simulink model "reglareperturbatie"  (R2016a)
settings: Solver=ode4  StartTime=0.0  StopTime=2000  FixedStep=0.01  RelTol=1e-3
undefined symbols (not defined in the file): k, k2, keta
libraries: simulink x1
settings Model: Creator=Danut  LastModifiedBy=Danut

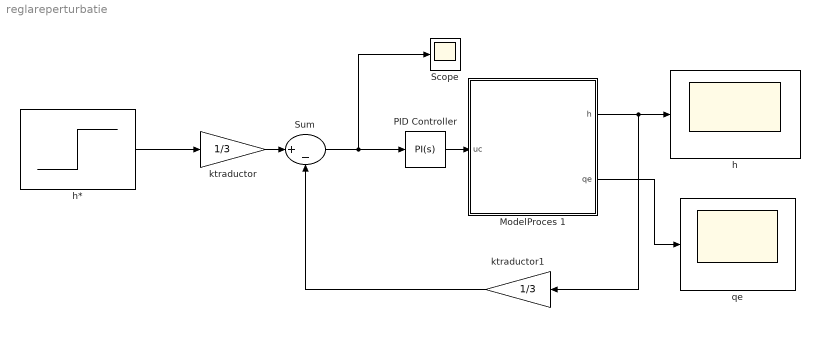
== system reglareperturbatie ==
  ModelProces 1 : Subsystem
  PID Controller : simulink/Continuous/PID Controller  Controller=PI  TimeDomain=Continuous-time  SampleTime=-1  IntegratorMethod=Forward Euler  FilterMethod=Forward Euler  Form=Parallel  UseFilter=on  ControllerParametersSource=internal  P=2.4  I=0.015  D=0  N=100  InitialConditionSource=internal  InitialConditionForIntegrator=5  InitialConditionForFilter=0  ExternalReset=none  LimitOutput=off  UpperSaturationLimit=inf  LowerSaturationLimit=-inf  LinearizeAsGain=on  AntiWindupMode=none  Kb=1  TrackingMode=off  Kt=1  PParamMin=[]  PParamMax=[]  IParamMin=[]  IParamMax=[]  DParamMin=[]  DParamMax=[]  NParamMin=[]  NParamMax=[]  KbParamMin=[]  KbParamMax=[]  KtParamMin=[]  KtParamMax=[]  POutMin=[]  POutMax=[]  IOutMin=[]  IOutMax=[]  DOutMin=[]  DOutMax=[]  NOutMin=[]  NOutMax=[]  KbOutMin=[]  KbOutMax=[]  KtOutMin=[]  KtOutMax=[]  IntegratorOutMin=[]  IntegratorOutMax=[]  FilterOutMin=[]  FilterOutMax=[]  SumOutMin=[]  SumOutMax=[]  SumI1OutMin=[]  SumI1OutMax=[]  SumI2OutMin=[]  SumI2OutMax=[]  SumI3OutMin=[]  SumI3OutMax=[]  SumDOutMin=[]  SumDOutMax=[]  SaturationOutMin=[]  SaturationOutMax=[]  IntegratorContinuousStateAttributes=''  IntegratorStateMustResolveToSignalObject=off  IntegratorRTWStateStorageClass=Auto  FilterContinuousStateAttributes=''  FilterStateMustResolveToSignalObject=off  FilterRTWStateStorageClass=Auto  DifferentiatorICPrevScaledInput=0  DifferentiatorOutMin=[]  DifferentiatorOutMax=[]
  Scope : Scope
  Sum : Sum  Inputs=|+-
  h : Scope
  h* : Step  Time=0  Before=10.5  After=13  SampleTime=0
  ktraductor : Gain  Gain=1/3
  ktraductor1 : Gain  Gain=1/3
  "qe " : Scope
  wires:
  ModelProces 1/1(h) -> ktraductor1/1, h/1
  ktraductor/1 -> Sum/1
  h*/1 -> ktraductor/1
  Sum/1 -> PID Controller/1, Scope/1
  ktraductor1/1 -> Sum/2
  PID Controller/1 -> ModelProces 1/1(uc)
  ModelProces 1/2(qe) -> "qe "/1

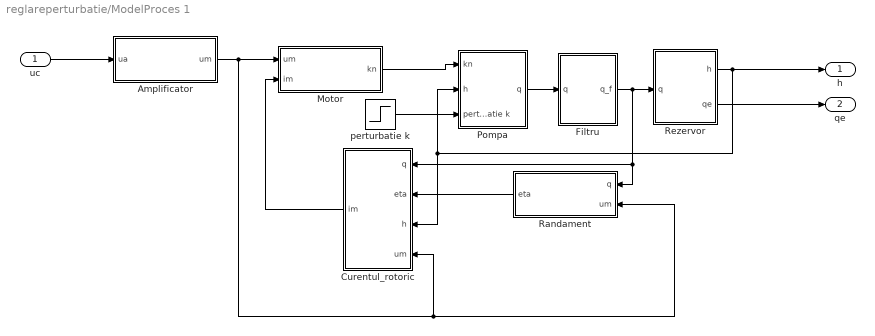
== system reglareperturbatie/ModelProces 1 ==
  uc : Inport
  "Amplificator " : Subsystem
  Curentul_rotoric : Subsystem
  Filtru : Subsystem
  "Motor " : Subsystem
  Pompa : Subsystem
  Randament : Subsystem
  Rezervor : Subsystem
  perturbatie k : Step  Time=1000  After=0.01  SampleTime=0
  h : Outport
  qe : Outport  Port=2
  wires:
  "Amplificator "/1("um ") -> "Motor "/1(um), Curentul_rotoric/4(um), Randament/2(um)
  "Motor "/1(kn) -> Pompa/1(kn)
  Pompa/1(q) -> Filtru/1(q)
  Filtru/1(q_f) -> Randament/1("q "), Curentul_rotoric/1(q), Rezervor/1(q)
  Rezervor/1(h) -> Curentul_rotoric/3(h), Pompa/2(h), h/1
  Curentul_rotoric/1(im) -> "Motor "/2(im)
  Randament/1("eta ") -> Curentul_rotoric/2(eta)
  uc/1 -> "Amplificator "/1(ua)
  Rezervor/2(qe) -> qe/1
  perturbatie k/1 -> Pompa/3(perturbatie k)

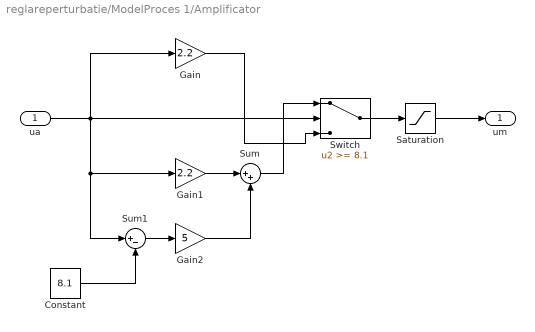
== system reglareperturbatie/ModelProces 1/Amplificator  ==
  ua : Inport
  Constant : Constant  Value=8.1
  Gain : Gain  Gain=2.2
  Gain1 : Gain  Gain=2.2
  Gain2 : Gain  Gain=5
  Saturation : Saturate  UpperLimit=22  LowerLimit=0
  Sum : Sum  Inputs=|++
  Sum1 : Sum  Inputs=|+-
  Switch : Switch  Threshold=8.1
  "um " : Outport
  wires:
  Sum1/1 -> Gain2/1
  ua/1 -> Switch/2, Gain/1, Sum1/1, Gain1/1
  Gain2/1 -> Sum/2
  Gain1/1 -> Sum/1
  Sum/1 -> Switch/1
  Gain/1 -> Switch/3
  Constant/1 -> Sum1/2
  Switch/1 -> Saturation/1
  Saturation/1 -> "um "/1

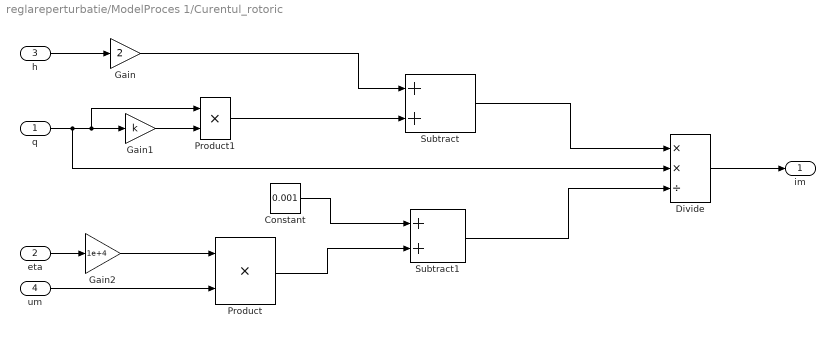
== system reglareperturbatie/ModelProces 1/Curentul_rotoric ==
  q : Inport
  eta : Inport  Port=2
  h : Inport  Port=3
  um : Inport  Port=4
  Constant : Constant  Value=0.001
  Divide : Product  Inputs=**/
  Gain : Gain  Gain=2
  Gain1 : Gain  Gain=k
  Gain2 : Gain  Gain=1e+4
  Product : Product
  Product1 : Product
  Subtract : Sum
  Subtract1 : Sum
  im : Outport
  wires:
  h/1 -> Gain/1
  Gain/1 -> Subtract/1
  q/1 -> Divide/2, Product1/1, Gain1/1
  Gain1/1 -> Product1/2
  Product1/1 -> Subtract/2
  eta/1 -> Gain2/1
  Gain2/1 -> Product/1
  um/1 -> Product/2
  Constant/1 -> Subtract1/1
  Product/1 -> Subtract1/2
  Divide/1 -> im/1
  Subtract/1 -> Divide/1
  Subtract1/1 -> Divide/3

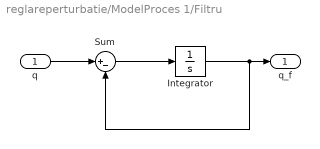
== system reglareperturbatie/ModelProces 1/Filtru ==
  q : Inport
  Integrator : Integrator  InitialCondition=29.2
  Sum : Sum  Inputs=|+-
  q_f : Outport
  wires:
  Integrator/1 -> Sum/2, q_f/1
  q/1 -> Sum/1
  Sum/1 -> Integrator/1

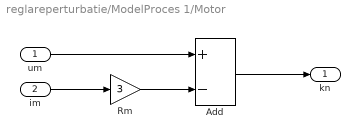
== system reglareperturbatie/ModelProces 1/Motor  ==
  um : Inport
  im : Inport  Port=2
  Add : Sum  Inputs=+-
  Rm : Gain  Gain=3
  kn : Outport
  wires:
  Rm/1 -> Add/2
  um/1 -> Add/1
  im/1 -> Rm/1
  Add/1 -> kn/1

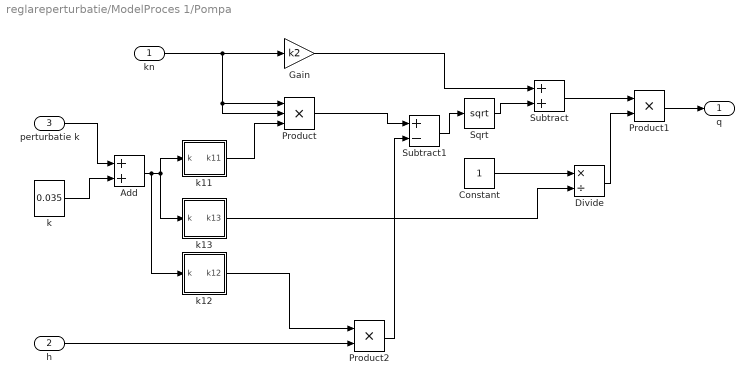
== system reglareperturbatie/ModelProces 1/Pompa ==
  kn : Inport
  h : Inport  Port=2
  perturbatie k : Inport  Port=3
  Add : Sum
  Constant : Constant
  Divide : Product  Inputs=*/
  Gain : Gain  Gain=k2
  Product : Product  Inputs=3
  Product1 : Product
  Product2 : Product
  Sqrt : Sqrt  SaturateOnIntegerOverflow=on
  Subtract : Sum
  Subtract1 : Sum  Inputs=+-
  "k " : Constant  Value=0.035
  "k11 " : Subsystem
  k12 : Subsystem
  k13 : Subsystem
  q : Outport
  wires:
  kn/1 -> Product/2, Product/1, Gain/1
  Sqrt/1 -> Subtract/2
  Gain/1 -> Subtract/1
  Subtract1/1 -> Sqrt/1
  Product/1 -> Subtract1/1
  Product1/1 -> q/1
  Subtract/1 -> Product1/1
  perturbatie k/1 -> Add/1
  "k "/1 -> Add/2
  h/1 -> Product2/2
  Add/1 -> k12/1(k), k13/1(k), "k11 "/1(k)
  "k11 "/1(k11) -> Product/3
  k12/1(k12) -> Product2/1
  Product2/1 -> Subtract1/2
  Constant/1 -> Divide/1
  k13/1(k13) -> Divide/2
  Divide/1 -> Product1/2

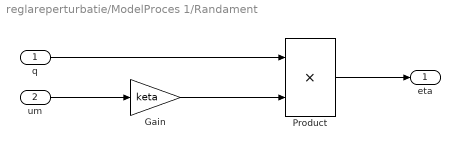
== system reglareperturbatie/ModelProces 1/Randament ==
  "q " : Inport
  um : Inport  Port=2
  Gain : Gain  Gain=keta
  Product : Product
  "eta " : Outport
  wires:
  um/1 -> Gain/1
  Gain/1 -> Product/2
  "q "/1 -> Product/1
  Product/1 -> "eta "/1

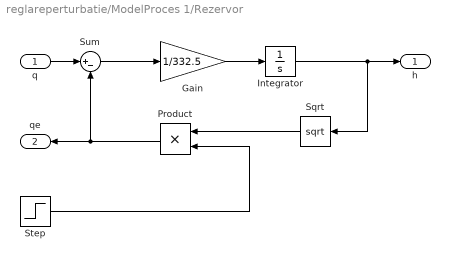
== system reglareperturbatie/ModelProces 1/Rezervor ==
  q : Inport
  Gain : Gain  Gain=1/332.5
  Integrator : Integrator  InitialCondition=10.5
  Product : Product
  Sqrt : Sqrt  SaturateOnIntegerOverflow=on
  Step : Step  Time=250  Before=9  After=11  SampleTime=0
  Sum : Sum  Inputs=|+-
  h : Outport
  qe : Outport  Port=2
  wires:
  Gain/1 -> Integrator/1
  Integrator/1 -> h/1, Sqrt/1
  q/1 -> Sum/1
  Sum/1 -> Gain/1
  Sqrt/1 -> Product/1
  Product/1 -> Sum/2, qe/1
  Step/1 -> Product/2

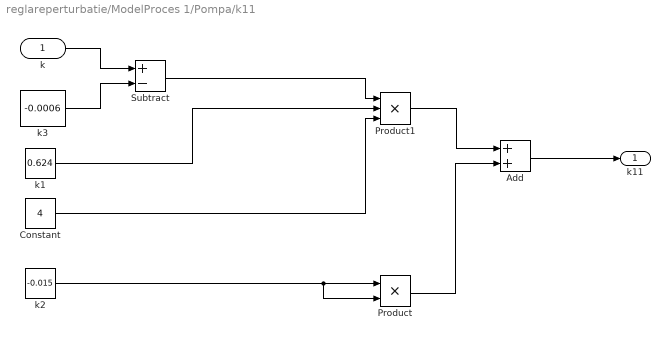
== system reglareperturbatie/ModelProces 1/Pompa/k11  ==
  k : Inport
  Add : Sum
  Constant : Constant  Value=4
  Product : Product
  Product1 : Product  Inputs=3
  Subtract : Sum  Inputs=+-
  k1 : Constant  Value=0.624
  k2 : Constant  Value=-0.015
  k3 : Constant  Value=-0.0006
  k11 : Outport
  wires:
  k2/1 -> Product/2, Product/1
  k/1 -> Subtract/1
  k3/1 -> Subtract/2
  Subtract/1 -> Product1/1
  k1/1 -> Product1/2
  Constant/1 -> Product1/3
  Product1/1 -> Add/1
  Product/1 -> Add/2
  Add/1 -> k11/1

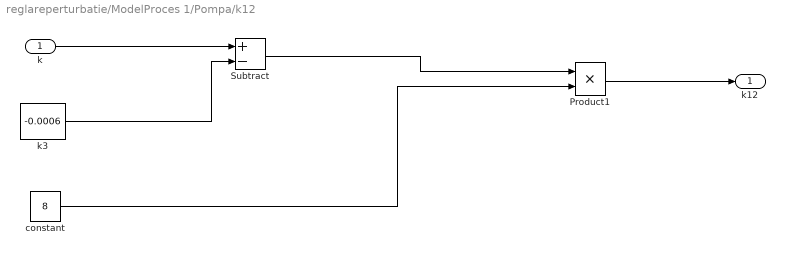
== system reglareperturbatie/ModelProces 1/Pompa/k12 ==
  k : Inport
  Product1 : Product
  Subtract : Sum  Inputs=+-
  "constant " : Constant  Value=8
  k3 : Constant  Value=-0.0006
  k12 : Outport
  wires:
  k/1 -> Subtract/1
  k3/1 -> Subtract/2
  Subtract/1 -> Product1/1
  "constant "/1 -> Product1/2
  Product1/1 -> k12/1

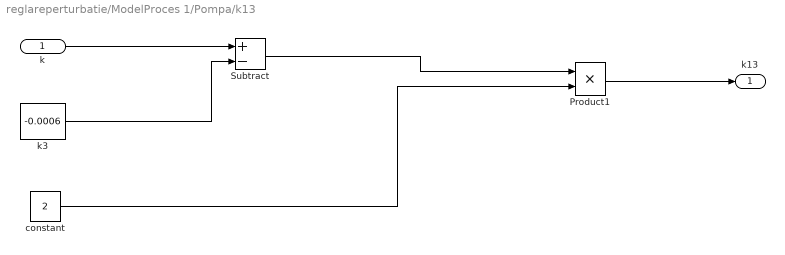
== system reglareperturbatie/ModelProces 1/Pompa/k13 ==
  k : Inport
  Product1 : Product
  Subtract : Sum  Inputs=+-
  "constant " : Constant  Value=2
  k3 : Constant  Value=-0.0006
  k13 : Outport
  wires:
  k/1 -> Subtract/1
  k3/1 -> Subtract/2
  Subtract/1 -> Product1/1
  "constant "/1 -> Product1/2
  Product1/1 -> k13/1
